simulink model "PID Simulation"  (R2022a)
settings: Solver=VariableStepAuto  StartTime=0.0  StopTime=10.0  RelTol=1e-3
undefined symbols (not defined in the file): tf1
libraries: simulink_extras x3, slpidlib x1, shared3dof x1, cstblocks x1
settings Model: Creator=rodri  LastModifiedBy=rodri

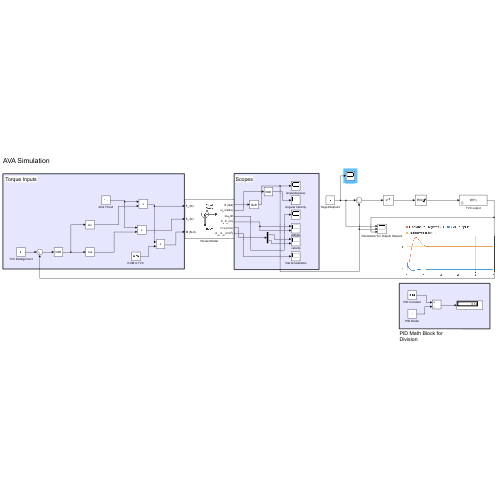
[thumbnail: Simulink's stored preview of the top-level diagram]
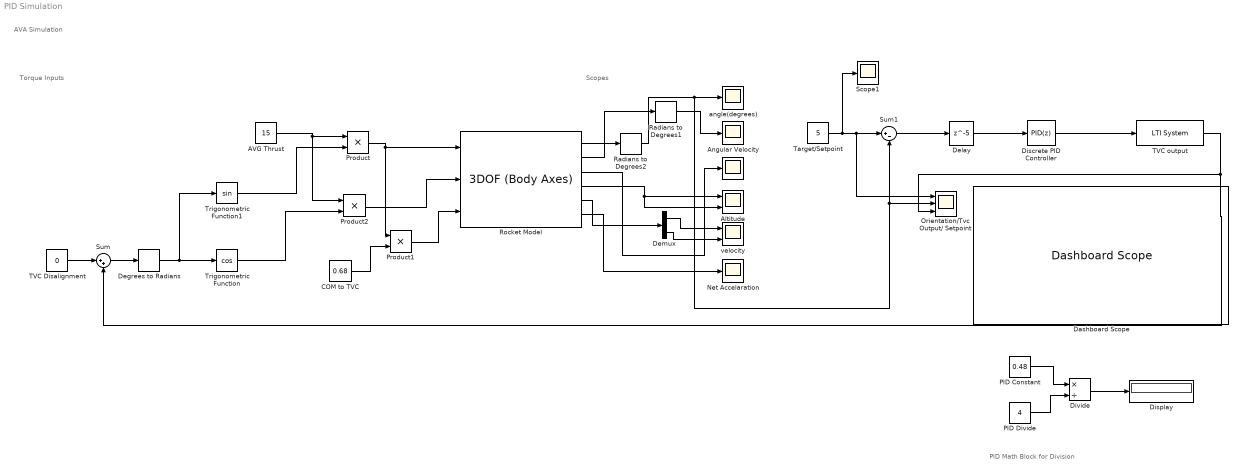
== system PID Simulation ==
  note: AVA Simulation
  note: Scopes
  note: Torque Inputs
  note: PID Math Block for Division
  " " : Scope
  " Altitude" : Scope  NumInputPorts=2
  " Net Accelaration" : Scope
  " velocity" : Scope  NumInputPorts=2
  AVG Thrust : Constant  Value=15
  Angular Velocity : Scope
  "COM to TVC " : Constant  Value=0.68
  Dashboard Scope : DashboardScope  ShowInitialText=off
  Degrees to Radians : simulink_extras/Transformations/Degrees to Radians
  Delay : Delay  DelayLength=5  InitialCondition=0
  Demux : Demux  Outputs=2
  Discrete PID Controller : slpidlib/PID Controller  Controller=PID  Form=Parallel  TimeDomain=Discrete-time  UseExternalTs=off  SampleTime=0.01  IntegratorMethod=Forward Euler  FilterMethod=Forward Euler  ControllerParametersSource=internal  P=0.14  I=0.12  UseKiTs=off  D=0.0575  N=100  UseFilter=off  TunerSelectOption=Transfer Function Based (PID Tuner App)  InitialConditionSource=internal  InitialConditionForIntegrator=0  InitialConditionForFilter=0  DifferentiatorICPrevScaledInput=0  ExternalReset=none  TrackingMode=off  Kt=1  LimitOutput=on  SatLimitsSource=internal  UpperSaturationLimit=5  LowerSaturationLimit=-5  LinearizeAsGain=off  AntiWindupMode=clamping  Kb=1  POutMin=[]  POutMax=[]  IOutMin=[]  IOutMax=[]  DOutMin=[]  DOutMax=[]  NOutMin=[]  NOutMax=[]  SumOutMin=[]  SumOutMax=[]  SaturationOutMin=[]  SaturationOutMax=[]  PParamMin=[]  PParamMax=[]  IParamMin=[]  IParamMax=[]  DParamMin=[]  DParamMax=[]  NParamMin=[]  NParamMax=[]  KbParamMin=[]  KbParamMax=[]  KtParamMin=[]  KtParamMax=[]  KbOutMin=[]  KbOutMax=[]  KtOutMin=[]  KtOutMax=[]  IntegratorOutMin=[]  IntegratorOutMax=[]  FilterOutMin=[]  FilterOutMax=[]  SumI1OutMin=[]  SumI1OutMax=[]  SumI2OutMin=[]  SumI2OutMax=[]  SumI3OutMin=[]  SumI3OutMax=[]  SumI4OutMin=[]  SumI4OutMax=[]  SumDOutMin=[]  SumDOutMax=[]  DifferentiatorOutMin=[]  DifferentiatorOutMax=[]  FilterDiffOutCoefMin=[]  FilterDiffOutCoefMax=[]  ReciprocalOutMin=[]  ReciprocalOutMax=[]  SumDenOutMin=[]  SumDenOutMax=[]  SumNumOutMin=[]  SumNumOutMax=[]  DivideOutMin=[]  DivideOutMax=[]  UdiffTsProdOutMin=[]  UdiffTsProdOutMax=[]  NTsProdOutMin=[]  NTsProdOutMax=[]  UintegralTsProdOutMin=[]  UintegralTsProdOutMax=[]  UngainTsProdOutMin=[]  UngainTsProdOutMax=[]  IntegratorContinuousStateAttributes=''  IntegratorStateMustResolveToSignalObject=off  IntegratorRTWStateStorageClass=Auto  FilterContinuousStateAttributes=''  FilterStateMustResolveToSignalObject=off  FilterRTWStateStorageClass=Auto  ParallelPVariant=InternalParameters  IdealPVariant=Disabled  IVariant=InternalParameters  DVariant=InternalParameters  IntegratorVariant=Discrete  SatVariant=Enabled  AWVariant=DiscClampingParallel  PCopyVariant=Disabled  TRVariant=Disabled  FdbkBlocksVariant=Forward  IdealPFdbkVariant=Disabled  SatFdbkVariant=Disabled  DerivativeFilterVariant=Differentiator  NVariant=Passthrough  NCopyVariant=Disabled_SignalSpec  FilterICVariant=InternalICsDifferentiator  IntegratorICVariant=InternalICs  ExternalResetVariant=Disabled  TRSumVariant=Passthrough  SumFdbkVariant=Disabled  SumVariant=Sum_PID  TsampFilterVariant=InternalTs  TsampNgainVariant=Passthrough  TsampIntegralVariant=Passthrough  ExternalSaturationOutDataTypeStr=Inherit: Same as second input  aMode=0
  Display : Display
  Divide : Product  Inputs=*/
  Orientation/Tvc Output/ Setpoint : Scope  NumInputPorts=3
  PID Constant : Constant  Value=0.48
  PID Divide : Constant  Value=4
  Product : Product
  Product1 : Product
  Product2 : Product
  Radians to Degrees1 : simulink_extras/Transformations/Radians to Degrees
  Radians to Degrees2 : simulink_extras/Transformations/Radians to Degrees
  Rocket Model : shared3dof/3DOF (Body Axes)  units=Metric (MKS)  mtype=Fixed  v_ini=0  theta_ini=0  alpha_ini=0  pos_ini=[0 0]  q_ini=0  mass=1.254  mass_e=0.5  mass_f=3.0  Iyy=0.128025  Iyy_e=0.5  Iyy_f=3.0  g_in=Internal  g=-9.81  vre_flag=on  abi_flag=off  aMode=0  vel_statename=''  theta_statename=''  pos_statename=''  q_statename=''  mass_statename=''
      settings: SourceProductBaseCode=AE,PW,DR,MT,VE
  Scope1 : Scope
  Sum : Sum  Inputs=|++
  Sum1 : Sum  Inputs=|+-
  TVC Disalignment : Constant  Value=0
  TVC output : cstblocks/LTI System  sys=tf(tf1)  IC=[]
  Target/Setpoint : Constant  Value=5
  Trigonometric Function : Trigonometry  Operator=cos
  Trigonometric Function1 : Trigonometry
  angle(degrees) : Scope
  wires:
  TVC Disalignment/1 -> Sum/1
  Rocket Model/1 -> Radians to Degrees2/1
  Target/Setpoint/1 -> Orientation/Tvc Output/ Setpoint/1, Sum1/1, Scope1/1
  Radians to Degrees2/1 -> Sum1/2, Orientation/Tvc Output/ Setpoint/2, angle(degrees)/1
  Discrete PID Controller/1 -> TVC output/1
  TVC output/1 -> Sum/2, Orientation/Tvc Output/ Setpoint/3
  Sum1/1 -> Delay/1
  Delay/1 -> Discrete PID Controller/1
  "COM to TVC "/1 -> Product1/2
  Product/1 -> Product1/1, Rocket Model/1
  Product1/1 -> Rocket Model/3
  AVG Thrust/1 -> Product/1, Product2/1
  Sum/1 -> Degrees to Radians/1
  Degrees to Radians/1 -> Trigonometric Function1/1, Trigonometric Function/1
  Trigonometric Function/1 -> Product2/2
  Trigonometric Function1/1 -> Product/2
  Product2/1 -> Rocket Model/2
  Rocket Model/2 -> Radians to Degrees1/1
  Radians to Degrees1/1 -> Angular Velocity/1
  Rocket Model/3 -> " "/1
  Rocket Model/4 -> " Altitude"/2, " Altitude"/1
  Rocket Model/6 -> " Net Accelaration"/1
  Rocket Model/5 -> Demux/1
  Demux/1 -> " velocity"/1
  Demux/2 -> " velocity"/2
  PID Constant/1 -> Divide/1
  PID Divide/1 -> Divide/2
  Divide/1 -> Display/1
